simulink model "rippleCarryAdderR2008a"  (Simulink 7.1)
settings: Solver=ode1  StartTime=0.0  StopTime=10.0  FixedStep=1  RelTol=1e-3
libraries: simulink x28, commutil2 x3
settings Model: Creator=Osmaz  LastModifiedBy=Osmaz
settings OptimizationCC: ExpressionDepthLimit=128  InitFltsAndDblsToZero=off
settings DebuggingCC: SolverPrmCheckMsg=none  FcnCallInpInsideContextMsg=Enable All  StateNameClashWarn=none  StrictBusMsg=ErrorLevel1
settings CodeAppCC: CustomSymbolStrType=$N$R$M_T
settings GRTTargetCC: TargetFunctionLibrary=C89/C90 (ANSI)  CPPClassGenCompliant=off
settings ConfigurationSet: Description=SimMechanics 2G

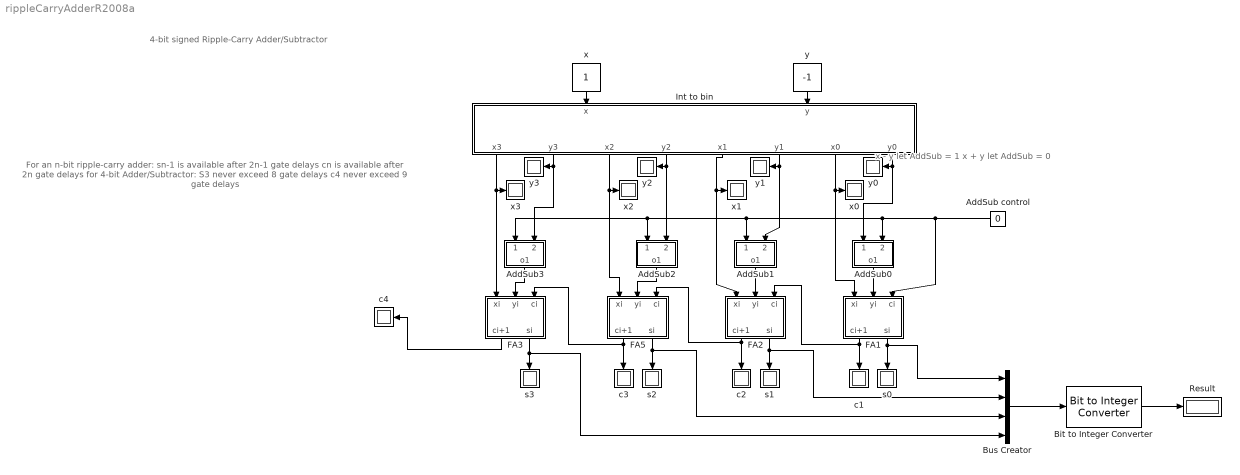
== system rippleCarryAdderR2008a ==
  note: For an n-bit ripple-carry adder:
      | sn-1 is available after 2n-1 gate delays
      | cn is available after 2n gate delays
      |
      | for 4-bit Adder/Subtractor:
      | S3 never exceed  8 gate delays
      | c4 never exceed 9 gate delays
  note: 4-bit signed Ripple-Carry Adder/Subtractor
  note: x - y let AddSub = 1
      | x + y let AddSub = 0
  AddSub control : Constant  Orientation=left  Value=0  OutMin=0  OutMax=1  OutDataTypeStr=boolean  OutDataTypeMode=boolean
  AddSub0 : Subsystem  Orientation=down
  AddSub1 : Subsystem  Orientation=down
  AddSub2 : Subsystem  Orientation=down
  AddSub3 : Subsystem  Orientation=down
  Bit to Integer Converter : commutil2/Bit to Integer Converter  nbits=4  bitOrder=LSB first  signedOutputValues=Signed  outDtype=Inherit via internal rule  outDtypeSigned=Inherit via internal rule
  Bus Creator : BusCreator
  FA1 : Subsystem  Orientation=down
  FA2 : Subsystem  Orientation=down
  FA3 : Subsystem  Orientation=down
  FA5 : Subsystem  Orientation=down
  Int to bin : Subsystem  Orientation=down
  Result : Display
  c{1..4} (4 alike) : Display
      c1 settings: Orientation=down
      c2 settings: Orientation=down
      c3 settings: Orientation=down
  s{0..3} (4 alike) : Display
      settings: Orientation=down
  x : Constant  Orientation=down  OutMin=-8  OutMax=7  OutDataTypeStr=int8  SampleTime=1  OutDataTypeMode=int8
  x{0..3} (4 alike) : Display
  y : Constant  Orientation=down  Value=-1  OutMin=-8  OutMax=7  OutDataTypeStr=int8  SampleTime=1  OutDataTypeMode=int8
  y{0..3} (4 alike) : Display
  wires:
  Int to bin/7(x0) -> x0/1, FA1/1(xi)
  AddSub control/1 -> FA1/3(ci), AddSub1/1(1), AddSub3/1(1), AddSub2/1(1), AddSub0/2(2)
  FA1/2(si) -> s0/1, Bus Creator/1
  Int to bin/5(x1) -> FA2/1(xi), x1/1
  FA2/2(si) -> Bus Creator/2, s1/1
  FA1/1(ci+1) -> FA2/3(ci), c1/1
  Int to bin/3(x2) -> FA5/1(xi), x2/1
  FA5/2(si) -> s2/1, Bus Creator/3
  FA2/1(ci+1) -> FA5/3(ci), c2/1
  Int to bin/1(x3) -> x3/1, FA3/1(xi)
  FA3/2(si) -> s3/1, Bus Creator/4
  FA5/1(ci+1) -> FA3/3(ci), c3/1
  FA3/1(ci+1) -> c4/1
  Bit to Integer Converter/1 -> Result/1
  Bus Creator/1 -> Bit to Integer Converter/1
  x/1 -> Int to bin/1(x)
  y/1 -> Int to bin/2(y)
  Int to bin/8(y0) -> AddSub0/1(1), y0/1
  Int to bin/6(y1) -> AddSub1/2(2), y1/1
  Int to bin/4(y2) -> y2/1, AddSub2/2(2)
  Int to bin/2(y3) -> AddSub3/2(2), y3/1
  AddSub1/1(o1) -> FA2/2(yi)
  AddSub2/1(o1) -> FA5/2(yi)
  AddSub3/1(o1) -> FA3/2(yi)
  AddSub0/1(o1) -> FA1/2(yi)

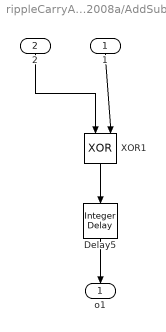
== system rippleCarryAdderR2008a/AddSub0 ==
  1 : Inport  Orientation=down
  2 : Inport  Orientation=down  Port=2
  Delay5 : simulink/Discrete/Integer Delay  Orientation=down  NumDelays=1  vinit=0  samptime=-1
  XOR1 : Logic  Orientation=down  Operator=XOR  IconShape=distinctive  AllPortsSameDT=off  OutDataTypeStr=boolean  OutDataTypeMode=boolean
  o1 : Outport  Orientation=down
  wires:
  1/1 -> XOR1/2
  2/1 -> XOR1/1
  XOR1/1 -> Delay5/1
  Delay5/1 -> o1/1

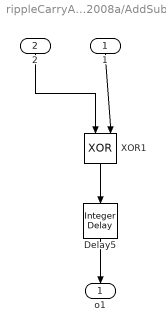
== system rippleCarryAdderR2008a/AddSub1 ==
  1 : Inport  Orientation=down
  2 : Inport  Orientation=down  Port=2
  Delay5 : simulink/Discrete/Integer Delay  Orientation=down  NumDelays=1  vinit=0  samptime=-1
  XOR1 : Logic  Orientation=down  Operator=XOR  IconShape=distinctive  AllPortsSameDT=off  OutDataTypeStr=boolean  OutDataTypeMode=boolean
  o1 : Outport  Orientation=down
  wires:
  1/1 -> XOR1/2
  2/1 -> XOR1/1
  XOR1/1 -> Delay5/1
  Delay5/1 -> o1/1

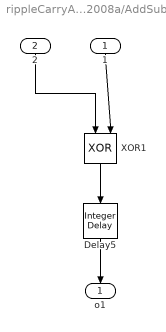
== system rippleCarryAdderR2008a/AddSub2 ==
  1 : Inport  Orientation=down
  2 : Inport  Orientation=down  Port=2
  Delay5 : simulink/Discrete/Integer Delay  Orientation=down  NumDelays=1  vinit=0  samptime=-1
  XOR1 : Logic  Orientation=down  Operator=XOR  IconShape=distinctive  AllPortsSameDT=off  OutDataTypeStr=boolean  OutDataTypeMode=boolean
  o1 : Outport  Orientation=down
  wires:
  1/1 -> XOR1/2
  2/1 -> XOR1/1
  XOR1/1 -> Delay5/1
  Delay5/1 -> o1/1

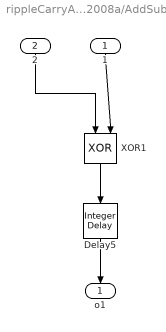
== system rippleCarryAdderR2008a/AddSub3 ==
  1 : Inport  Orientation=down
  2 : Inport  Orientation=down  Port=2
  Delay5 : simulink/Discrete/Integer Delay  Orientation=down  NumDelays=1  vinit=0  samptime=-1
  XOR1 : Logic  Orientation=down  Operator=XOR  IconShape=distinctive  AllPortsSameDT=off  OutDataTypeStr=boolean  OutDataTypeMode=boolean
  o1 : Outport  Orientation=down
  wires:
  1/1 -> XOR1/2
  2/1 -> XOR1/1
  XOR1/1 -> Delay5/1
  Delay5/1 -> o1/1

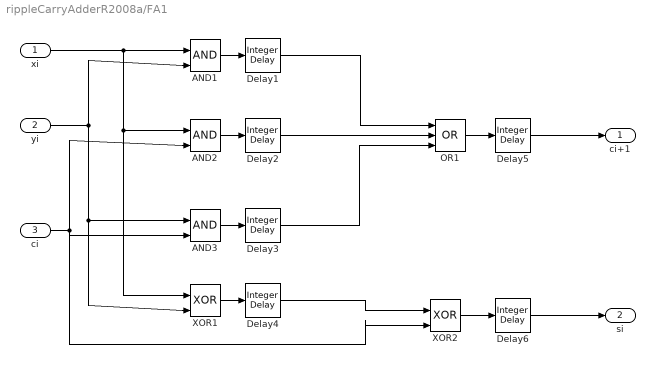
== system rippleCarryAdderR2008a/FA1 ==
  xi : Inport
  yi : Inport  Port=2
  ci : Inport  Port=3
  AND1 : Logic  IconShape=distinctive  AllPortsSameDT=off  OutDataTypeStr=boolean  OutDataTypeMode=boolean
  AND2 : Logic  IconShape=distinctive  AllPortsSameDT=off  OutDataTypeStr=boolean  OutDataTypeMode=boolean
  AND3 : Logic  IconShape=distinctive  AllPortsSameDT=off  OutDataTypeStr=boolean  OutDataTypeMode=boolean
  Delay{1..6} (6 alike) : simulink/Discrete/Integer Delay  NumDelays=1  vinit=0  samptime=-1
  OR1 : Logic  Operator=OR  Inputs=3  IconShape=distinctive  AllPortsSameDT=off  OutDataTypeStr=boolean  OutDataTypeMode=boolean
  XOR1 : Logic  Operator=XOR  IconShape=distinctive  AllPortsSameDT=off  OutDataTypeStr=boolean  OutDataTypeMode=boolean
  XOR2 : Logic  Operator=XOR  IconShape=distinctive  AllPortsSameDT=off  OutDataTypeStr=boolean  OutDataTypeMode=boolean
  ci+1 : Outport
  si : Outport  Port=2
  wires:
  Delay1/1 -> OR1/1
  AND1/1 -> Delay1/1
  yi/1 -> AND1/2, XOR1/2, AND3/1
  xi/1 -> AND1/1, XOR1/1, AND2/1
  AND2/1 -> Delay2/1
  Delay2/1 -> OR1/2
  AND3/1 -> Delay3/1
  Delay3/1 -> OR1/3
  ci/1 -> XOR2/2, AND2/2, AND3/2
  OR1/1 -> Delay5/1
  Delay5/1 -> ci+1/1
  Delay6/1 -> si/1
  XOR1/1 -> Delay4/1
  Delay4/1 -> XOR2/1
  XOR2/1 -> Delay6/1

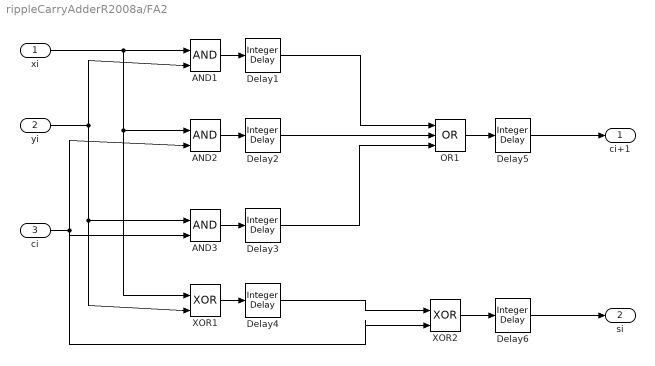
== system rippleCarryAdderR2008a/FA2 ==
  xi : Inport
  yi : Inport  Port=2
  ci : Inport  Port=3
  AND1 : Logic  IconShape=distinctive  AllPortsSameDT=off  OutDataTypeStr=boolean  OutDataTypeMode=boolean
  AND2 : Logic  IconShape=distinctive  AllPortsSameDT=off  OutDataTypeStr=boolean  OutDataTypeMode=boolean
  AND3 : Logic  IconShape=distinctive  AllPortsSameDT=off  OutDataTypeStr=boolean  OutDataTypeMode=boolean
  Delay{1..6} (6 alike) : simulink/Discrete/Integer Delay  NumDelays=1  vinit=0  samptime=-1
  OR1 : Logic  Operator=OR  Inputs=3  IconShape=distinctive  AllPortsSameDT=off  OutDataTypeStr=boolean  OutDataTypeMode=boolean
  XOR1 : Logic  Operator=XOR  IconShape=distinctive  AllPortsSameDT=off  OutDataTypeStr=boolean  OutDataTypeMode=boolean
  XOR2 : Logic  Operator=XOR  IconShape=distinctive  AllPortsSameDT=off  OutDataTypeStr=boolean  OutDataTypeMode=boolean
  ci+1 : Outport
  si : Outport  Port=2
  wires:
  Delay1/1 -> OR1/1
  AND1/1 -> Delay1/1
  yi/1 -> AND1/2, XOR1/2, AND3/1
  xi/1 -> AND1/1, XOR1/1, AND2/1
  AND2/1 -> Delay2/1
  Delay2/1 -> OR1/2
  AND3/1 -> Delay3/1
  Delay3/1 -> OR1/3
  ci/1 -> XOR2/2, AND2/2, AND3/2
  OR1/1 -> Delay5/1
  Delay5/1 -> ci+1/1
  Delay6/1 -> si/1
  XOR1/1 -> Delay4/1
  Delay4/1 -> XOR2/1
  XOR2/1 -> Delay6/1

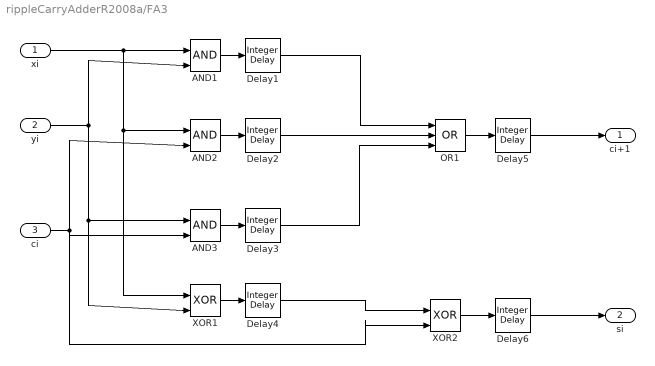
== system rippleCarryAdderR2008a/FA3 ==
  xi : Inport
  yi : Inport  Port=2
  ci : Inport  Port=3
  AND1 : Logic  IconShape=distinctive  AllPortsSameDT=off  OutDataTypeStr=boolean  OutDataTypeMode=boolean
  AND2 : Logic  IconShape=distinctive  AllPortsSameDT=off  OutDataTypeStr=boolean  OutDataTypeMode=boolean
  AND3 : Logic  IconShape=distinctive  AllPortsSameDT=off  OutDataTypeStr=boolean  OutDataTypeMode=boolean
  Delay{1..6} (6 alike) : simulink/Discrete/Integer Delay  NumDelays=1  vinit=0  samptime=-1
  OR1 : Logic  Operator=OR  Inputs=3  IconShape=distinctive  AllPortsSameDT=off  OutDataTypeStr=boolean  OutDataTypeMode=boolean
  XOR1 : Logic  Operator=XOR  IconShape=distinctive  AllPortsSameDT=off  OutDataTypeStr=boolean  OutDataTypeMode=boolean
  XOR2 : Logic  Operator=XOR  IconShape=distinctive  AllPortsSameDT=off  OutDataTypeStr=boolean  OutDataTypeMode=boolean
  ci+1 : Outport
  si : Outport  Port=2
  wires:
  Delay1/1 -> OR1/1
  AND1/1 -> Delay1/1
  yi/1 -> AND1/2, XOR1/2, AND3/1
  xi/1 -> AND1/1, XOR1/1, AND2/1
  AND2/1 -> Delay2/1
  Delay2/1 -> OR1/2
  AND3/1 -> Delay3/1
  Delay3/1 -> OR1/3
  ci/1 -> XOR2/2, AND2/2, AND3/2
  OR1/1 -> Delay5/1
  Delay5/1 -> ci+1/1
  Delay6/1 -> si/1
  XOR1/1 -> Delay4/1
  Delay4/1 -> XOR2/1
  XOR2/1 -> Delay6/1

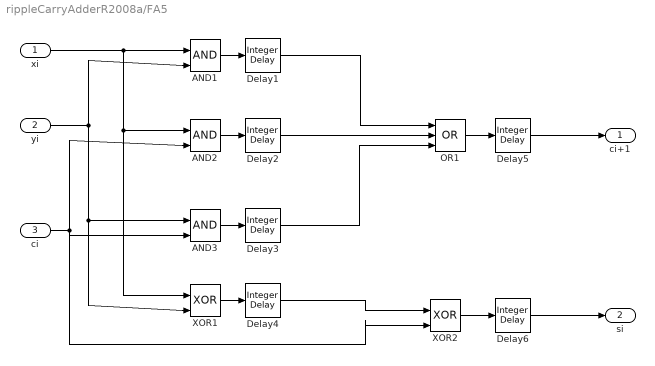
== system rippleCarryAdderR2008a/FA5 ==
  xi : Inport
  yi : Inport  Port=2
  ci : Inport  Port=3
  AND1 : Logic  IconShape=distinctive  AllPortsSameDT=off  OutDataTypeStr=boolean  OutDataTypeMode=boolean
  AND2 : Logic  IconShape=distinctive  AllPortsSameDT=off  OutDataTypeStr=boolean  OutDataTypeMode=boolean
  AND3 : Logic  IconShape=distinctive  AllPortsSameDT=off  OutDataTypeStr=boolean  OutDataTypeMode=boolean
  Delay{1..6} (6 alike) : simulink/Discrete/Integer Delay  NumDelays=1  vinit=0  samptime=-1
  OR1 : Logic  Operator=OR  Inputs=3  IconShape=distinctive  AllPortsSameDT=off  OutDataTypeStr=boolean  OutDataTypeMode=boolean
  XOR1 : Logic  Operator=XOR  IconShape=distinctive  AllPortsSameDT=off  OutDataTypeStr=boolean  OutDataTypeMode=boolean
  XOR2 : Logic  Operator=XOR  IconShape=distinctive  AllPortsSameDT=off  OutDataTypeStr=boolean  OutDataTypeMode=boolean
  ci+1 : Outport
  si : Outport  Port=2
  wires:
  Delay1/1 -> OR1/1
  AND1/1 -> Delay1/1
  yi/1 -> AND1/2, XOR1/2, AND3/1
  xi/1 -> AND1/1, XOR1/1, AND2/1
  AND2/1 -> Delay2/1
  Delay2/1 -> OR1/2
  AND3/1 -> Delay3/1
  Delay3/1 -> OR1/3
  ci/1 -> XOR2/2, AND2/2, AND3/2
  OR1/1 -> Delay5/1
  Delay5/1 -> ci+1/1
  Delay6/1 -> si/1
  XOR1/1 -> Delay4/1
  Delay4/1 -> XOR2/1
  XOR2/1 -> Delay6/1

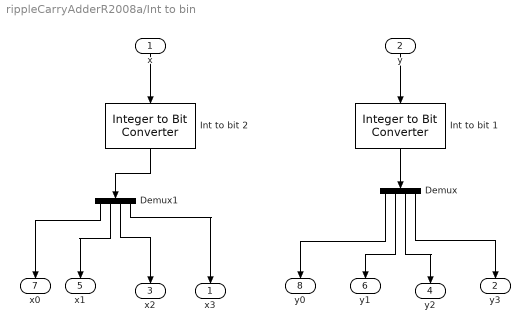
== system rippleCarryAdderR2008a/Int to bin ==
  x : Inport  Orientation=down
  y : Inport  Orientation=down  Port=2
  Demux : Demux  Orientation=down
  Demux1 : Demux  Orientation=down
  Int to bit 1 : commutil2/Integer to Bit Converter  Orientation=down  nbits=4  signedInputValues=Signed  bitOrder=LSB first  outDtype=Inherit via internal rule
  Int to bit 2 : commutil2/Integer to Bit Converter  Orientation=down  nbits=4  signedInputValues=Signed  bitOrder=LSB first  outDtype=Inherit via internal rule
  x3 : Outport  Orientation=down
  y3 : Outport  Orientation=down  Port=2
  x2 : Outport  Orientation=down  Port=3
  y2 : Outport  Orientation=down  Port=4
  x1 : Outport  Orientation=down  Port=5
  y1 : Outport  Orientation=down  Port=6
  x0 : Outport  Orientation=down  Port=7
  y0 : Outport  Orientation=down  Port=8
  wires:
  Demux1/1 -> x0/1
  Demux/2 -> y1/1
  Demux1/2 -> x1/1
  Demux/1 -> y0/1
  y/1 -> Int to bit 1/1
  Int to bit 1/1 -> Demux/1
  x/1 -> Int to bit 2/1
  Demux1/3 -> x2/1
  Demux1/4 -> x3/1
  Demux/3 -> y2/1
  Int to bit 2/1 -> Demux1/1
  Demux/4 -> y3/1
